simulink model "physic_mods_2state"  (Simulink 7.8)
settings: Solver=ode3  StartTime=0.0  StopTime=time_span  FixedStep=samp_time  RelTol=1e-3
values from neighbouring files (symbols this model uses):
  IC = rand(2,1)    [simulate_ode.m]
  outstr = {'10*(u(2)-(1/3*(u(1)^3-u(1))))'    [simulate_ode.m]
  samp_time = 0.1    [simulate_ode.m]
settings Model: Creator=TheQuarry  LastModifiedBy=TheQuarry

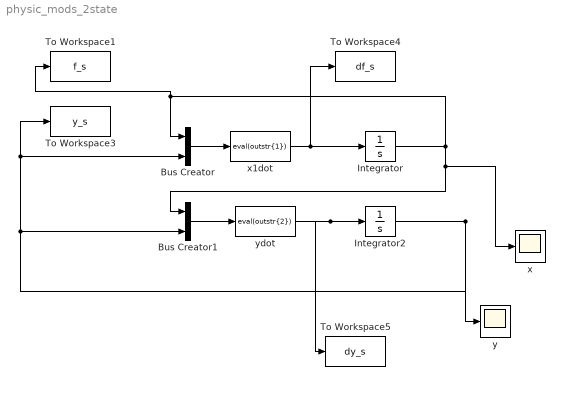
== system physic_mods_2state ==
  Bus Creator : BusCreator  Inputs=2
  Bus Creator1 : BusCreator  Inputs=2
  Integrator : Integrator  InitialCondition=IC(1)
  Integrator2 : Integrator  InitialCondition=IC(2)
  To Workspace1 : ToWorkspace  VariableName=f_s  SampleTime=-1  SaveFormat=Array
  To Workspace3 : ToWorkspace  VariableName=y_s  SampleTime=-1  SaveFormat=Array
  To Workspace4 : ToWorkspace  VariableName=df_s  SampleTime=-1  SaveFormat=Array
  To Workspace5 : ToWorkspace  VariableName=dy_s  SampleTime=-1  SaveFormat=Array
  x : Scope
  x1dot : MATLABFcn  MATLABFcn=eval(outstr{1})  SampleTime=samp_time
  y : Scope
  ydot : MATLABFcn  MATLABFcn=eval(outstr{2})
  wires:
  Bus Creator/1 -> x1dot/1
  Bus Creator1/1 -> ydot/1
  Integrator/1 -> Bus Creator/1, To Workspace1/1, Bus Creator1/1, x/1
  Integrator2/1 -> Bus Creator/2, To Workspace3/1, Bus Creator1/2, y/1
  x1dot/1 -> Integrator/1, To Workspace4/1
  ydot/1 -> Integrator2/1, To Workspace5/1
